simulink model "ControlPC_lab2"  (R2015a)
settings: Solver=ode45  StartTime=0.0  StopTime=10.0  RelTol=1e-3
values from neighbouring files (symbols this model uses):
  beta = 0.065    [parametros.m]    (also in ploteo.m)
  J = 0.02    [parametros.m]    (also in ploteo.m)
  Kf = 20    [parametros.m]    (also in ploteo.m)
  Kpe = 0.26    [parametros.m]    (also in ploteo.m)
  Kpi = 0.014    [parametros.m]    (also in ploteo.m)
  T = 0.04    [parametros.m]    (also in ploteo.m)
  tau = 0.2    [parametros.m]    (also in ploteo.m)
  Ti = 0.25    [parametros.m]    (also in ploteo.m)
settings Model: Creator=ARTURO  LastModifiedBy=ARTURO

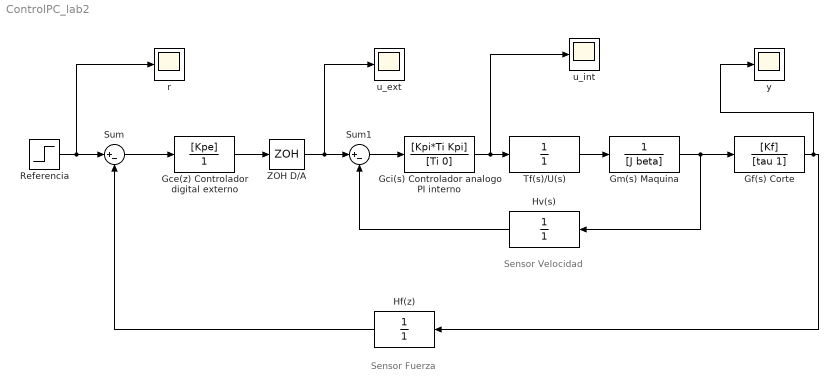
== system ControlPC_lab2 ==
  note: Sensor Fuerza
  note: Sensor Velocidad
  " Hf(z) " : DiscreteTransferFcn  Denominator=[1]  SampleTime=T
  Gce(z) Controlador digital externo : DiscreteTransferFcn  Numerator=[Kpe]  Denominator=[1]  SampleTime=T
  Gci(s) Controlador analogo PI interno : TransferFcn  Numerator=[Kpi*Ti Kpi]  Denominator=[Ti 0]
  Gf(s) Corte : TransferFcn  Numerator=[Kf]  Denominator=[tau 1]
  Gm(s) Maquina : TransferFcn  Denominator=[J beta]
  Hv(s) : TransferFcn  Denominator=[1]
  Referencia : Step  SampleTime=T
  Sum : Sum  Inputs=|+-
  Sum1 : Sum  Inputs=|+-
  Tf(s)/U(s) : TransferFcn  Denominator=[1]
  ZOH D/A : ZeroOrderHold  SampleTime=T
  "r " : Scope
      settings: SaveName=r
  u_ext : Scope
      settings: SaveName=u
  "u_int " : Scope
      settings: SaveName=u_int
  "y " : Scope
      settings: SaveName=y
  wires:
  Sum/1 -> Gce(z) Controlador digital externo/1
  Referencia/1 -> "r "/1, Sum/1
  Gce(z) Controlador digital externo/1 -> ZOH D/A/1
  ZOH D/A/1 -> u_ext/1, Sum1/1
  Sum1/1 -> Gci(s) Controlador analogo PI interno/1
  Gci(s) Controlador analogo PI interno/1 -> "u_int "/1, Tf(s)/U(s)/1
  Tf(s)/U(s)/1 -> Gm(s) Maquina/1
  Gm(s) Maquina/1 -> Hv(s)/1, Gf(s) Corte/1
  Hv(s)/1 -> Sum1/2
  Gf(s) Corte/1 -> "y "/1, " Hf(z) "/1
  " Hf(z) "/1 -> Sum/2
